simulink model "AircraftModel_LonMot"  (R2020b)
settings: Solver=VariableStepAuto  StartTime=0.0  StopTime=150  FixedStep=CNT_StepSize  RelTol=1e-3
values from neighbouring files (symbols this model uses):
  CNT_g = 9.81    [AircraftParameters_LonMot.m]
  CNT_m = 15917    [AircraftParameters_LonMot.m]
undefined symbols (not defined in the file or in its folder): Propulsion
libraries: vrlib x2
settings Model: Creator=NicolasS  LastModifiedBy=vlsag
settings DataIOCC: ExternalInput=getinputstruct(report1)  InitialState=getstatestruct(report1)

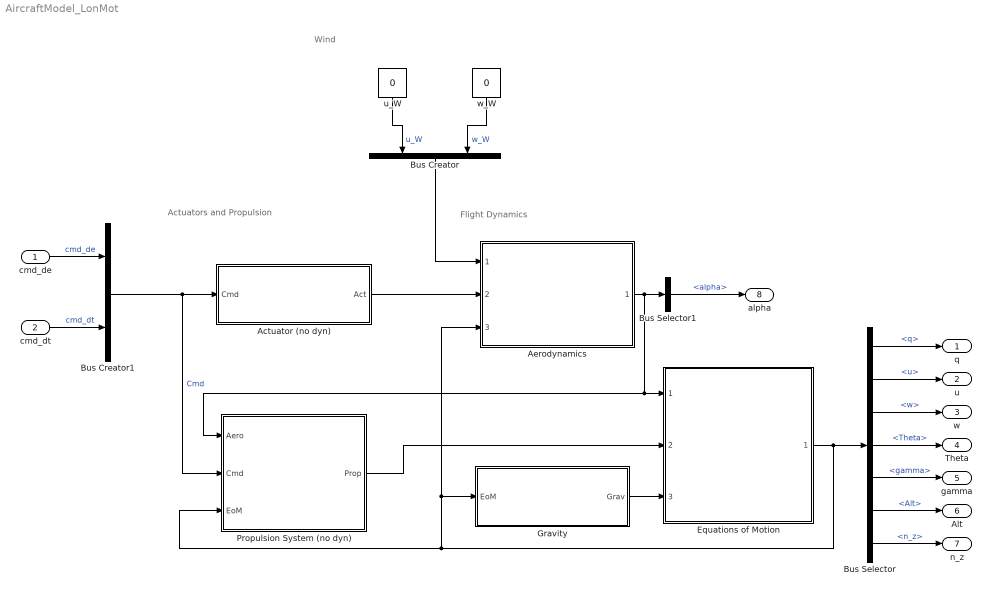
== system AircraftModel_LonMot ==
  note: Wind
  note: Actuators and Propulsion
  note: Flight Dynamics
  cmd_de : Inport
  cmd_dt : Inport  Port=2
  Actuator (no dyn) : Subsystem
  Aerodynamics : Subsystem  ReferencedSubsystem=Aerodyn
  Bus Creator : BusCreator  Inputs=2  OutDataTypeStr=Bus: WaT
  Bus Creator1 : BusCreator  Inputs=2  OutDataTypeStr=Bus: Cmd
  Bus Selector : BusSelector  OutputSignals=q,vv_f.u,vv_f.w,Theta,gamma,Alt,nn_f.n_z
  Bus Selector1 : BusSelector  OutputSignals=AirData.alpha
  Equations of Motion : Subsystem  ReferencedSubsystem=Equations_of_Motion
  Gravity : Subsystem
  Propulsion System (no dyn) : Subsystem
  u_W : Constant  Value=0  SampleTime=-1
  w_W : Constant  Value=0  SampleTime=-1
  q : Outport
  u : Outport  Port=2
  w : Outport  Port=3
  Theta : Outport  Port=4
  gamma : Outport  Port=5
  Alt : Outport  Port=6
  n_z : Outport  Port=7
  alpha : Outport  Port=8
  wires:
  cmd_de/1 -> Bus Creator1/1  "cmd_de"
  cmd_dt/1 -> Bus Creator1/2  "cmd_dt"
  u_W/1 -> Bus Creator/1  "u_W"
  Actuator (no dyn)/1(Act) -> Aerodynamics/2
  Aerodynamics/1 -> Bus Selector1/1, Propulsion System (no dyn)/1(Aero), Equations of Motion/1
  w_W/1 -> Bus Creator/2  "w_W"
  Equations of Motion/1 -> Propulsion System (no dyn)/3(EoM), Aerodynamics/3, Gravity/1(EoM), Bus Selector/1
  Bus Creator1/1 -> Actuator (no dyn)/1(Cmd), Propulsion System (no dyn)/2(Cmd)  "Cmd"
  Propulsion System (no dyn)/1(Prop) -> Equations of Motion/2
  Bus Selector/6 -> Alt/1  "<Alt>"
  Bus Selector/1 -> q/1  "<q>"
  Bus Selector/2 -> u/1  "<u>"
  Bus Selector/3 -> w/1  "<w>"
  Bus Selector/4 -> Theta/1  "<Theta>"
  Bus Selector/7 -> n_z/1  "<n_z>"
  Bus Selector1/1 -> alpha/1  "<alpha>"
  Gravity/1(Grav) -> Equations of Motion/3
  Bus Selector/5 -> gamma/1  "<gamma>"
  Bus Creator/1 -> Aerodynamics/1

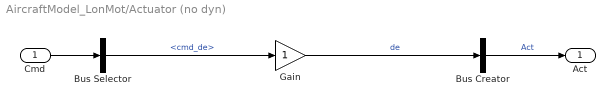
== system AircraftModel_LonMot/Actuator (no dyn) ==
  Cmd : Inport  OutDataTypeStr=Bus: Cmd
  Bus Creator : BusCreator  Inputs=1  OutDataTypeStr=Bus: Act
  Bus Selector : BusSelector  OutputSignals=cmd_de
  Gain : Gain
  Act : Outport  OutDataTypeStr=Bus: Act
  wires:
  Bus Creator/1 -> Act/1  "Act"
  Cmd/1 -> Bus Selector/1
  Gain/1 -> Bus Creator/1  "de"
  Bus Selector/1 -> Gain/1  "<cmd_de>"

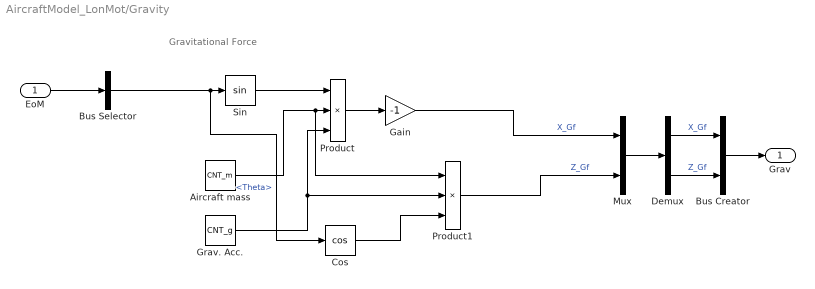
== system AircraftModel_LonMot/Gravity ==
  note: Gravitational Force
  EoM : Inport  OutDataTypeStr=Bus: EoM
  Aircraft mass : Constant  Value=CNT_m  SampleTime=-1
  Bus Creator : BusCreator  Inputs=2  OutDataTypeStr=Bus: Grav
  Bus Selector : BusSelector  OutputSignals=Theta
  Cos : Trigonometry  Operator=cos
  Demux : Demux  Outputs=2
  Gain : Gain  Gain=-1
  Grav. Acc. : Constant  Value=CNT_g  SampleTime=-1
  Mux : Mux  Inputs=2
  Product : Product  Inputs=3
  Product1 : Product  Inputs=3
  Sin : Trigonometry
  Grav : Outport  OutDataTypeStr=Bus: Grav
  wires:
  EoM/1 -> Bus Selector/1
  Demux/1 -> Bus Creator/1  "X_Gf"
  Demux/2 -> Bus Creator/2  "Z_Gf"
  Bus Creator/1 -> Grav/1
  Mux/1 -> Demux/1
  Bus Selector/1 -> Cos/1, Sin/1  "<Theta>"
  Sin/1 -> Product/1
  Aircraft mass/1 -> Product1/1, Product/2
  Grav. Acc./1 -> Product1/2, Product/3
  Product/1 -> Gain/1
  Gain/1 -> Mux/1  "X_Gf"
  Cos/1 -> Product1/3
  Product1/1 -> Mux/2  "Z_Gf"

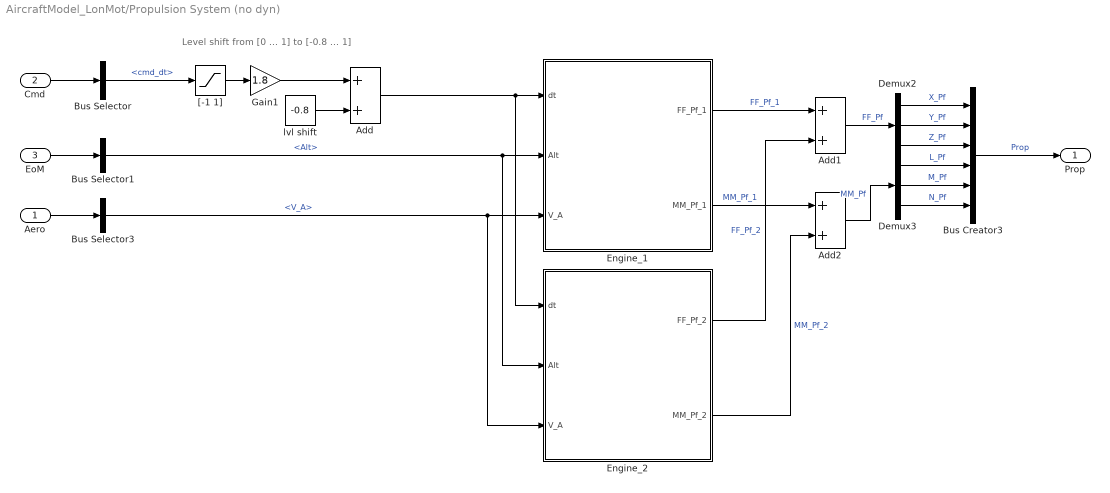
== system AircraftModel_LonMot/Propulsion System (no dyn) ==
  note: Level shift from [0 ... 1] to [-0.8 ... 1]
  Aero : Inport  OutDataTypeStr=Bus: Aero
  Cmd : Inport  Port=2  OutDataTypeStr=Bus: Cmd
  EoM : Inport  Port=3  OutDataTypeStr=Bus: EoM
  Add : Sum
  Add1 : Sum
  Add2 : Sum
  Bus Creator3 : BusCreator  Inputs=6  OutDataTypeStr=Bus: Prop
  Bus Selector : BusSelector  OutputSignals=cmd_dt
  Bus Selector1 : BusSelector  OutputSignals=Alt
  Bus Selector3 : BusSelector  OutputSignals=AirData.V_A
  Demux2 : Demux  Outputs=3
  Demux3 : Demux  Outputs=3
  Engine_1 : Subsystem
  Engine_2 : Subsystem
  Gain1 : Gain  Gain=1.8
  "[-1 1]" : Saturate  UpperLimit=1  LowerLimit=0
  lvl shift : Constant  Value=-0.8  SampleTime=-1
  Prop : Outport  OutDataTypeStr=Bus: Prop
  wires:
  Demux2/2 -> Bus Creator3/2  "Y_Pf"
  Engine_1/1(FF_Pf_1) -> Add1/1  "FF_Pf_1"
  Demux3/1 -> Bus Creator3/4  "L_Pf"
  EoM/1 -> Bus Selector1/1
  lvl shift/1 -> Add/2
  Engine_2/1(FF_Pf_2) -> Add1/2  "FF_Pf_2"
  Add2/1 -> Demux3/1  "MM_Pf"
  Bus Selector3/1 -> Engine_2/3(V_A), Engine_1/3(V_A)  "<V_A>"
  Aero/1 -> Bus Selector3/1
  Demux2/1 -> Bus Creator3/1  "X_Pf"
  Gain1/1 -> Add/1
  Engine_1/2(MM_Pf_1) -> Add2/1  "MM_Pf_1"
  Add/1 -> Engine_2/1(dt), Engine_1/1(dt)
  Bus Creator3/1 -> Prop/1  "Prop"
  Demux3/2 -> Bus Creator3/5  "M_Pf"
  "[-1 1]"/1 -> Gain1/1
  Demux2/3 -> Bus Creator3/3  "Z_Pf"
  Add1/1 -> Demux2/1  "FF_Pf"
  Bus Selector1/1 -> Engine_2/2(Alt), Engine_1/2(Alt)  "<Alt>"
  Demux3/3 -> Bus Creator3/6  "N_Pf"
  Cmd/1 -> Bus Selector/1
  Bus Selector/1 -> "[-1 1]"/1  "<cmd_dt>"
  Engine_2/2(MM_Pf_2) -> Add2/2  "MM_Pf_2"

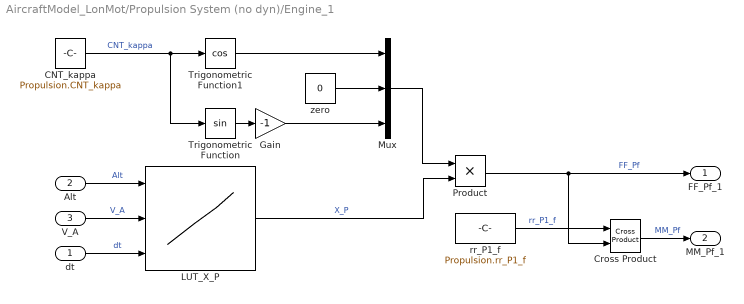
== system AircraftModel_LonMot/Propulsion System (no dyn)/Engine_1 ==
  dt : Inport
  Alt : Inport  Port=2
  V_A : Inport  Port=3
  CNT_kappa : Constant  Value=Propulsion.CNT_kappa  SampleTime=-1
  Cross Product : vrlib/Utilities/Cross Product
  Gain : Gain  Gain=-1
  LUT_X_P : Lookup_n-D  NumberOfTableDimensions=3  BreakpointsForDimension1=Propulsion.LUT.LUT_Alt  BreakpointsForDimension2=Propulsion.LUT.LUT_V_A  BreakpointsForDimension3=Propulsion.LUT.LUT_dt  Table=Propulsion.LUT.LUT_X_P  ExtrapMethod=Clip  InputSameDT=on
      settings: InputPortMap=u0,u1,u2
  Mux : Mux  Inputs=3
  Product : Product  RndMeth=Zero
  Trigonometric Function : Trigonometry
  Trigonometric Function1 : Trigonometry  Operator=cos
  "rr_P1_f " : Constant  Value=Propulsion.rr_P1_f  SampleTime=-1
  zero : Constant  Value=0  SampleTime=-1
  FF_Pf_1 : Outport
  MM_Pf_1 : Outport  Port=2
  wires:
  Alt/1 -> LUT_X_P/1  "Alt"
  V_A/1 -> LUT_X_P/2  "V_A"
  dt/1 -> LUT_X_P/3  "dt"
  zero/1 -> Mux/2
  Mux/1 -> Product/1
  CNT_kappa/1 -> Trigonometric Function1/1, Trigonometric Function/1  "CNT_kappa"
  Trigonometric Function1/1 -> Mux/1
  Product/1 -> FF_Pf_1/1, Cross Product/2  "FF_Pf"
  Cross Product/1 -> MM_Pf_1/1  "MM_Pf"
  Trigonometric Function/1 -> Gain/1
  Gain/1 -> Mux/3
  LUT_X_P/1 -> Product/2  "X_P"
  "rr_P1_f "/1 -> Cross Product/1  "rr_P1_f"

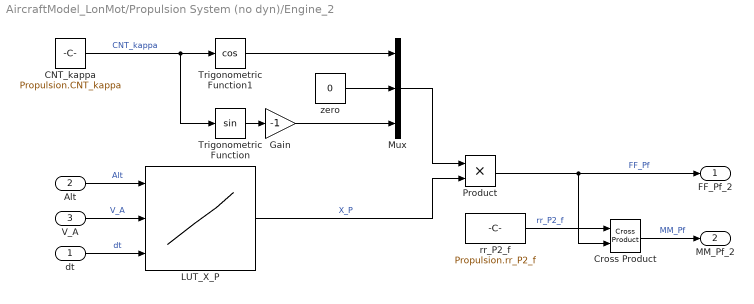
== system AircraftModel_LonMot/Propulsion System (no dyn)/Engine_2 ==
  dt : Inport
  Alt : Inport  Port=2
  V_A : Inport  Port=3
  CNT_kappa : Constant  Value=Propulsion.CNT_kappa  SampleTime=-1
  Cross Product : vrlib/Utilities/Cross Product
  Gain : Gain  Gain=-1
  LUT_X_P : Lookup_n-D  NumberOfTableDimensions=3  BreakpointsForDimension1=Propulsion.LUT.LUT_Alt  BreakpointsForDimension2=Propulsion.LUT.LUT_V_A  BreakpointsForDimension3=Propulsion.LUT.LUT_dt  Table=Propulsion.LUT.LUT_X_P  InputSameDT=on
      settings: InputPortMap=u0,u1,u2
  Mux : Mux  Inputs=3
  Product : Product  RndMeth=Zero
  Trigonometric Function : Trigonometry
  Trigonometric Function1 : Trigonometry  Operator=cos
  "rr_P2_f " : Constant  Value=Propulsion.rr_P2_f  SampleTime=-1
  zero : Constant  Value=0  SampleTime=-1
  FF_Pf_2 : Outport
  MM_Pf_2 : Outport  Port=2
  wires:
  zero/1 -> Mux/2
  Gain/1 -> Mux/3
  Mux/1 -> Product/1
  Cross Product/1 -> MM_Pf_2/1  "MM_Pf"
  Trigonometric Function1/1 -> Mux/1
  Product/1 -> FF_Pf_2/1, Cross Product/2  "FF_Pf"
  Trigonometric Function/1 -> Gain/1
  Alt/1 -> LUT_X_P/1  "Alt"
  dt/1 -> LUT_X_P/3  "dt"
  LUT_X_P/1 -> Product/2  "X_P"
  V_A/1 -> LUT_X_P/2  "V_A"
  "rr_P2_f "/1 -> Cross Product/1  "rr_P2_f"
  CNT_kappa/1 -> Trigonometric Function1/1, Trigonometric Function/1  "CNT_kappa"
